simulink model "DriveSystemControl"  (R2023b)
settings: Solver=FixedStepAuto  StartTime=0.0  StopTime=Inf  FixedStep=0.001  RelTol=1e-3
PostLoadFcn:
  | if any(exist('dsrtsu_mdlpostloadfcn', 'file') ~= 0), dsrtsu_mdlpostloadfcn('Execute', bdroot); end
InitFcn:
  | , if any(exist('rtifpga_mdlclblib', 'file') ~= 0), rtifpga_mdlclblib('Init', bdroot); end,
  | , if any(exist('dsmpb_private', 'file') ~= 0), dsmpb_private('dsmpb_mdlclblib', 'Init', bdroot); end,
libraries: dsmpblib x2
(part 9 of 11)

== system DriveSystemControl/Bus Configuration (1) - Out/Manipulation/Virya Controller CAN File 08082024/WIP/CANChannel/PDUs/BMS02/sigBatteryCurrent/Feature Switch ==
  Feature Switch : Inport
  Term_sigBatteryCurrent Current Countdown Value : Terminator
  Term_sigBatteryCurrent Selected Feature : Terminator
  _Feature Switch_ : BusSelector  OutputSignals=sigBatteryCurrent Current Countdown Value,sigBatteryCurrent Selected Feature
  wires:
  Feature Switch/1 -> _Feature Switch_/1  "Feature Switch"
  _Feature Switch_/1 -> Term_sigBatteryCurrent Current Countdown Value/1  "<sigBatteryCurrent Current Countdown Value>"
  _Feature Switch_/2 -> Term_sigBatteryCurrent Selected Feature/1  "<sigBatteryCurrent Selected Feature>"

== system DriveSystemControl/Bus Configuration (1) - Out/Manipulation/Virya Controller CAN File 08082024/WIP/CANChannel/PDUs/BMS02/sigDriveCurrentLimit/Feature Switch ==
  Feature Switch : Inport
  Term_sigDriveCurrentLimit Current Countdown Value : Terminator
  Term_sigDriveCurrentLimit Selected Feature : Terminator
  _Feature Switch_ : BusSelector  OutputSignals=sigDriveCurrentLimit Current Countdown Value,sigDriveCurrentLimit Selected Feature
  wires:
  Feature Switch/1 -> _Feature Switch_/1  "Feature Switch"
  _Feature Switch_/1 -> Term_sigDriveCurrentLimit Current Countdown Value/1  "<sigDriveCurrentLimit Current Countdown Value>"
  _Feature Switch_/2 -> Term_sigDriveCurrentLimit Selected Feature/1  "<sigDriveCurrentLimit Selected Feature>"

== system DriveSystemControl/Bus Configuration (1) - Out/Manipulation/Virya Controller CAN File 08082024/WIP/CANChannel/PDUs/BMS02/sigRegenCurrentLimit/Feature Switch ==
  Feature Switch : Inport
  Term_sigRegenCurrentLimit Current Countdown Value : Terminator
  Term_sigRegenCurrentLimit Selected Feature : Terminator
  _Feature Switch_ : BusSelector  OutputSignals=sigRegenCurrentLimit Current Countdown Value,sigRegenCurrentLimit Selected Feature
  wires:
  Feature Switch/1 -> _Feature Switch_/1  "Feature Switch"
  _Feature Switch_/1 -> Term_sigRegenCurrentLimit Current Countdown Value/1  "<sigRegenCurrentLimit Current Countdown Value>"
  _Feature Switch_/2 -> Term_sigRegenCurrentLimit Selected Feature/1  "<sigRegenCurrentLimit Selected Feature>"

== system DriveSystemControl/Bus Configuration (1) - Out/Manipulation/Virya Controller CAN File 08082024/WIP/CANChannel/PDUs/BMS02/sigVehicleModeRequest/Feature Switch ==
  Feature Switch : Inport
  Term_sigVehicleModeRequest Current Countdown Value : Terminator
  Term_sigVehicleModeRequest Selected Feature : Terminator
  _Feature Switch_ : BusSelector  OutputSignals=sigVehicleModeRequest Current Countdown Value,sigVehicleModeRequest Selected Feature
  wires:
  Feature Switch/1 -> _Feature Switch_/1  "Feature Switch"
  _Feature Switch_/1 -> Term_sigVehicleModeRequest Current Countdown Value/1  "<sigVehicleModeRequest Current Countdown Value>"
  _Feature Switch_/2 -> Term_sigVehicleModeRequest Selected Feature/1  "<sigVehicleModeRequest Selected Feature>"

== system DriveSystemControl/Bus Configuration (1) - Out/Manipulation/Virya Controller CAN File 08082024/WIP/CANChannel/PDUs/MainController/CCU_heartBeat/Feature Switch ==
  Feature Switch : Inport
  Term_CCU_heartBeat Current Countdown Value : Terminator
  Term_CCU_heartBeat Selected Feature : Terminator
  _Feature Switch_ : BusSelector  OutputSignals=CCU_heartBeat Current Countdown Value,CCU_heartBeat Selected Feature
  wires:
  Feature Switch/1 -> _Feature Switch_/1  "Feature Switch"
  _Feature Switch_/1 -> Term_CCU_heartBeat Current Countdown Value/1  "<CCU_heartBeat Current Countdown Value>"
  _Feature Switch_/2 -> Term_CCU_heartBeat Selected Feature/1  "<CCU_heartBeat Selected Feature>"

== system DriveSystemControl/Bus Configuration (1) - Out/Manipulation/Virya Controller CAN File 08082024/WIP/CANChannel/PDUs/MainController/notUsed/Feature Switch ==
  Feature Switch : Inport
  Term_notUsed Current Countdown Value : Terminator
  Term_notUsed Selected Feature : Terminator
  _Feature Switch_ : BusSelector  OutputSignals=notUsed Current Countdown Value,notUsed Selected Feature
  wires:
  Feature Switch/1 -> _Feature Switch_/1  "Feature Switch"
  _Feature Switch_/1 -> Term_notUsed Current Countdown Value/1  "<notUsed Current Countdown Value>"
  _Feature Switch_/2 -> Term_notUsed Selected Feature/1  "<notUsed Selected Feature>"

== system DriveSystemControl/Bus Configuration (1) - Out/Manipulation/Virya Controller CAN File 08082024/WIP/CANChannel/PDUs/MainController/setAutoParkBreak/Feature Switch ==
  Feature Switch : Inport
  Term_setAutoParkBreak Current Countdown Value : Terminator
  Term_setAutoParkBreak Selected Feature : Terminator
  _Feature Switch_ : BusSelector  OutputSignals=setAutoParkBreak Current Countdown Value,setAutoParkBreak Selected Feature
  wires:
  Feature Switch/1 -> _Feature Switch_/1  "Feature Switch"
  _Feature Switch_/1 -> Term_setAutoParkBreak Current Countdown Value/1  "<setAutoParkBreak Current Countdown Value>"
  _Feature Switch_/2 -> Term_setAutoParkBreak Selected Feature/1  "<setAutoParkBreak Selected Feature>"

== system DriveSystemControl/Bus Configuration (1) - Out/Manipulation/Virya Controller CAN File 08082024/WIP/CANChannel/PDUs/MainController/setBreake/Feature Switch ==
  Feature Switch : Inport
  Term_setBreake Current Countdown Value : Terminator
  Term_setBreake Selected Feature : Terminator
  _Feature Switch_ : BusSelector  OutputSignals=setBreake Current Countdown Value,setBreake Selected Feature
  wires:
  Feature Switch/1 -> _Feature Switch_/1  "Feature Switch"
  _Feature Switch_/1 -> Term_setBreake Current Countdown Value/1  "<setBreake Current Countdown Value>"
  _Feature Switch_/2 -> Term_setBreake Selected Feature/1  "<setBreake Selected Feature>"

== system DriveSystemControl/Bus Configuration (1) - Out/Manipulation/Virya Controller CAN File 08082024/WIP/CANChannel/PDUs/MainController/setDirection/Feature Switch ==
  Feature Switch : Inport
  Term_setDirection Current Countdown Value : Terminator
  Term_setDirection Selected Feature : Terminator
  _Feature Switch_ : BusSelector  OutputSignals=setDirection Current Countdown Value,setDirection Selected Feature
  wires:
  Feature Switch/1 -> _Feature Switch_/1  "Feature Switch"
  _Feature Switch_/1 -> Term_setDirection Current Countdown Value/1  "<setDirection Current Countdown Value>"
  _Feature Switch_/2 -> Term_setDirection Selected Feature/1  "<setDirection Selected Feature>"

== system DriveSystemControl/Bus Configuration (1) - Out/Manipulation/Virya Controller CAN File 08082024/WIP/CANChannel/PDUs/MainController/setDriveMode/Feature Switch ==
  Feature Switch : Inport
  Term_setDriveMode Current Countdown Value : Terminator
  Term_setDriveMode Selected Feature : Terminator
  _Feature Switch_ : BusSelector  OutputSignals=setDriveMode Current Countdown Value,setDriveMode Selected Feature
  wires:
  Feature Switch/1 -> _Feature Switch_/1  "Feature Switch"
  _Feature Switch_/1 -> Term_setDriveMode Current Countdown Value/1  "<setDriveMode Current Countdown Value>"
  _Feature Switch_/2 -> Term_setDriveMode Selected Feature/1  "<setDriveMode Selected Feature>"

== system DriveSystemControl/Bus Configuration (1) - Out/Manipulation/Virya Controller CAN File 08082024/WIP/CANChannel/PDUs/MainController/setVelocity/Feature Switch ==
  Feature Switch : Inport
  Term_setVelocity Current Countdown Value : Terminator
  Term_setVelocity Selected Feature : Terminator
  _Feature Switch_ : BusSelector  OutputSignals=setVelocity Current Countdown Value,setVelocity Selected Feature
  wires:
  Feature Switch/1 -> _Feature Switch_/1  "Feature Switch"
  _Feature Switch_/1 -> Term_setVelocity Current Countdown Value/1  "<setVelocity Current Countdown Value>"
  _Feature Switch_/2 -> Term_setVelocity Selected Feature/1  "<setVelocity Selected Feature>"

== system DriveSystemControl/Bus Configuration (1) - Out/Manipulation/Virya Controller CAN File 08082024/WIP/CANChannel/PDUs/MainController/steeringPower/Feature Switch ==
  Feature Switch : Inport
  Term_steeringPower Current Countdown Value : Terminator
  Term_steeringPower Selected Feature : Terminator
  _Feature Switch_ : BusSelector  OutputSignals=steeringPower Current Countdown Value,steeringPower Selected Feature
  wires:
  Feature Switch/1 -> _Feature Switch_/1  "Feature Switch"
  _Feature Switch_/1 -> Term_steeringPower Current Countdown Value/1  "<steeringPower Current Countdown Value>"
  _Feature Switch_/2 -> Term_steeringPower Selected Feature/1  "<steeringPower Selected Feature>"

== system DriveSystemControl/Bus Configuration (1) - Out/Manipulation/Virya Controller CAN File 08082024/WIP/CANChannel/PDUs/TCU01/sigBrake/Feature Switch ==
  Feature Switch : Inport
  Term_sigBrake Current Countdown Value : Terminator
  Term_sigBrake Selected Feature : Terminator
  _Feature Switch_ : BusSelector  OutputSignals=sigBrake Current Countdown Value,sigBrake Selected Feature
  wires:
  Feature Switch/1 -> _Feature Switch_/1  "Feature Switch"
  _Feature Switch_/1 -> Term_sigBrake Current Countdown Value/1  "<sigBrake Current Countdown Value>"
  _Feature Switch_/2 -> Term_sigBrake Selected Feature/1  "<sigBrake Selected Feature>"

== system DriveSystemControl/Bus Configuration (1) - Out/Manipulation/Virya Controller CAN File 08082024/WIP/CANChannel/PDUs/TCU01/sigControllerTemperature/Feature Switch ==
  Feature Switch : Inport
  Term_sigControllerTemperature Current Countdown Value : Terminator
  Term_sigControllerTemperature Selected Feature : Terminator
  _Feature Switch_ : BusSelector  OutputSignals=sigControllerTemperature Current Countdown Value,sigControllerTemperature Selected Feature
  wires:
  Feature Switch/1 -> _Feature Switch_/1  "Feature Switch"
  _Feature Switch_/1 -> Term_sigControllerTemperature Current Countdown Value/1  "<sigControllerTemperature Current Countdown Value>"
  _Feature Switch_/2 -> Term_sigControllerTemperature Selected Feature/1  "<sigControllerTemperature Selected Feature>"

== system DriveSystemControl/Bus Configuration (1) - Out/Manipulation/Virya Controller CAN File 08082024/WIP/CANChannel/PDUs/TCU01/sigDriveMode/Feature Switch ==
  Feature Switch : Inport
  Term_sigDriveMode Current Countdown Value : Terminator
  Term_sigDriveMode Selected Feature : Terminator
  _Feature Switch_ : BusSelector  OutputSignals=sigDriveMode Current Countdown Value,sigDriveMode Selected Feature
  wires:
  Feature Switch/1 -> _Feature Switch_/1  "Feature Switch"
  _Feature Switch_/1 -> Term_sigDriveMode Current Countdown Value/1  "<sigDriveMode Current Countdown Value>"
  _Feature Switch_/2 -> Term_sigDriveMode Selected Feature/1  "<sigDriveMode Selected Feature>"

== system DriveSystemControl/Bus Configuration (1) - Out/Manipulation/Virya Controller CAN File 08082024/WIP/CANChannel/PDUs/TCU01/sigMotorTemperature/Feature Switch ==
  Feature Switch : Inport
  Term_sigMotorTemperature Current Countdown Value : Terminator
  Term_sigMotorTemperature Selected Feature : Terminator
  _Feature Switch_ : BusSelector  OutputSignals=sigMotorTemperature Current Countdown Value,sigMotorTemperature Selected Feature
  wires:
  Feature Switch/1 -> _Feature Switch_/1  "Feature Switch"
  _Feature Switch_/1 -> Term_sigMotorTemperature Current Countdown Value/1  "<sigMotorTemperature Current Countdown Value>"
  _Feature Switch_/2 -> Term_sigMotorTemperature Selected Feature/1  "<sigMotorTemperature Selected Feature>"

== system DriveSystemControl/Bus Configuration (1) - Out/Manipulation/Virya Controller CAN File 08082024/WIP/CANChannel/PDUs/TCU01/sigRMSCurrent/Feature Switch ==
  Feature Switch : Inport
  Term_sigRMSCurrent Current Countdown Value : Terminator
  Term_sigRMSCurrent Selected Feature : Terminator
  _Feature Switch_ : BusSelector  OutputSignals=sigRMSCurrent Current Countdown Value,sigRMSCurrent Selected Feature
  wires:
  Feature Switch/1 -> _Feature Switch_/1  "Feature Switch"
  _Feature Switch_/1 -> Term_sigRMSCurrent Current Countdown Value/1  "<sigRMSCurrent Current Countdown Value>"
  _Feature Switch_/2 -> Term_sigRMSCurrent Selected Feature/1  "<sigRMSCurrent Selected Feature>"

== system DriveSystemControl/Bus Configuration (1) - Out/Manipulation/Virya Controller CAN File 08082024/WIP/CANChannel/PDUs/TCU01/sigSpeed/Feature Switch ==
  Feature Switch : Inport
  Term_sigSpeed Current Countdown Value : Terminator
  Term_sigSpeed Selected Feature : Terminator
  _Feature Switch_ : BusSelector  OutputSignals=sigSpeed Current Countdown Value,sigSpeed Selected Feature
  wires:
  Feature Switch/1 -> _Feature Switch_/1  "Feature Switch"
  _Feature Switch_/1 -> Term_sigSpeed Current Countdown Value/1  "<sigSpeed Current Countdown Value>"
  _Feature Switch_/2 -> Term_sigSpeed Selected Feature/1  "<sigSpeed Selected Feature>"

== system DriveSystemControl/Bus Configuration (1) - Out/Manipulation/Virya Controller CAN File 08082024/WIP/CANChannel/PDUs/TCU01/sigThrottle/Feature Switch ==
  Feature Switch : Inport
  Term_sigThrottle Current Countdown Value : Terminator
  Term_sigThrottle Selected Feature : Terminator
  _Feature Switch_ : BusSelector  OutputSignals=sigThrottle Current Countdown Value,sigThrottle Selected Feature
  wires:
  Feature Switch/1 -> _Feature Switch_/1  "Feature Switch"
  _Feature Switch_/1 -> Term_sigThrottle Current Countdown Value/1  "<sigThrottle Current Countdown Value>"
  _Feature Switch_/2 -> Term_sigThrottle Selected Feature/1  "<sigThrottle Selected Feature>"

== system DriveSystemControl/Bus Configuration (1) - Out/Manipulation/Virya Controller CAN File 08082024/WIP/CANChannel/PDUs/TCU02/sigCapacitorVoltage/Feature Switch ==
  Feature Switch : Inport
  Term_sigCapacitorVoltage Current Countdown Value : Terminator
  Term_sigCapacitorVoltage Selected Feature : Terminator
  _Feature Switch_ : BusSelector  OutputSignals=sigCapacitorVoltage Current Countdown Value,sigCapacitorVoltage Selected Feature
  wires:
  Feature Switch/1 -> _Feature Switch_/1  "Feature Switch"
  _Feature Switch_/1 -> Term_sigCapacitorVoltage Current Countdown Value/1  "<sigCapacitorVoltage Current Countdown Value>"
  _Feature Switch_/2 -> Term_sigCapacitorVoltage Selected Feature/1  "<sigCapacitorVoltage Selected Feature>"

== system DriveSystemControl/Bus Configuration (1) - Out/Manipulation/Virya Controller CAN File 08082024/WIP/CANChannel/PDUs/TCU02/sigMotorRPM/Feature Switch ==
  Feature Switch : Inport
  Term_sigMotorRPM Current Countdown Value : Terminator
  Term_sigMotorRPM Selected Feature : Terminator
  _Feature Switch_ : BusSelector  OutputSignals=sigMotorRPM Current Countdown Value,sigMotorRPM Selected Feature
  wires:
  Feature Switch/1 -> _Feature Switch_/1  "Feature Switch"
  _Feature Switch_/1 -> Term_sigMotorRPM Current Countdown Value/1  "<sigMotorRPM Current Countdown Value>"
  _Feature Switch_/2 -> Term_sigMotorRPM Selected Feature/1  "<sigMotorRPM Selected Feature>"

== system DriveSystemControl/Bus Configuration (1) - Out/Manipulation/Virya Controller CAN File 08082024/WIP/CANChannel/PDUs/TCU02/sigOdometer/Feature Switch ==
  Feature Switch : Inport
  Term_sigOdometer Current Countdown Value : Terminator
  Term_sigOdometer Selected Feature : Terminator
  _Feature Switch_ : BusSelector  OutputSignals=sigOdometer Current Countdown Value,sigOdometer Selected Feature
  wires:
  Feature Switch/1 -> _Feature Switch_/1  "Feature Switch"
  _Feature Switch_/1 -> Term_sigOdometer Current Countdown Value/1  "<sigOdometer Current Countdown Value>"
  _Feature Switch_/2 -> Term_sigOdometer Selected Feature/1  "<sigOdometer Selected Feature>"

== system DriveSystemControl/Bus Configuration (1) - Out/Manipulation/Virya Controller CAN File 08082024/WIP/CANChannel/PDUs/TCU03/Controller_CompleteFaults/Feature Switch ==
  Feature Switch : Inport
  Term_Controller_CompleteFaults Current Countdown Value : Terminator
  Term_Controller_CompleteFaults Selected Feature : Terminator
  _Feature Switch_ : BusSelector  OutputSignals=Controller_CompleteFaults Current Countdown Value,Controller_CompleteFaults Selected Feature
  wires:
  Feature Switch/1 -> _Feature Switch_/1  "Feature Switch"
  _Feature Switch_/1 -> Term_Controller_CompleteFaults Current Countdown Value/1  "<Controller_CompleteFaults Current Countdown Value>"
  _Feature Switch_/2 -> Term_Controller_CompleteFaults Selected Feature/1  "<Controller_CompleteFaults Selected Feature>"

== system DriveSystemControl/Bus Configuration (1) - Out/Manipulation/Virya Controller CAN File 08082024/WIP/CANChannel/PDUs/TCU03/sig5VSupplyFailure/Feature Switch ==
  Feature Switch : Inport
  Term_sig5VSupplyFailure Current Countdown Value : Terminator
  Term_sig5VSupplyFailure Selected Feature : Terminator
  _Feature Switch_ : BusSelector  OutputSignals=sig5VSupplyFailure Current Countdown Value,sig5VSupplyFailure Selected Feature
  wires:
  Feature Switch/1 -> _Feature Switch_/1  "Feature Switch"
  _Feature Switch_/1 -> Term_sig5VSupplyFailure Current Countdown Value/1  "<sig5VSupplyFailure Current Countdown Value>"
  _Feature Switch_/2 -> Term_sig5VSupplyFailure Selected Feature/1  "<sig5VSupplyFailure Selected Feature>"

== system DriveSystemControl/Bus Configuration (1) - Out/Manipulation/Virya Controller CAN File 08082024/WIP/CANChannel/PDUs/TCU03/sigBPosOvervoltageCutback/Feature Switch ==
  Feature Switch : Inport
  Term_sigBPosOvervoltageCutback Current Countdown Value : Terminator
  Term_sigBPosOvervoltageCutback Selected Feature : Terminator
  _Feature Switch_ : BusSelector  OutputSignals=sigBPosOvervoltageCutback Current Countdown Value,sigBPosOvervoltageCutback Selected Feature
  wires:
  Feature Switch/1 -> _Feature Switch_/1  "Feature Switch"
  _Feature Switch_/1 -> Term_sigBPosOvervoltageCutback Current Countdown Value/1  "<sigBPosOvervoltageCutback Current Countdown Value>"
  _Feature Switch_/2 -> Term_sigBPosOvervoltageCutback Selected Feature/1  "<sigBPosOvervoltageCutback Selected Feature>"

== system DriveSystemControl/Bus Configuration (1) - Out/Manipulation/Virya Controller CAN File 08082024/WIP/CANChannel/PDUs/TCU03/sigBPosUndervoltageCutback/Feature Switch ==
  Feature Switch : Inport
  Term_sigBPosUndervoltageCutback Current Countdown Value : Terminator
  Term_sigBPosUndervoltageCutback Selected Feature : Terminator
  _Feature Switch_ : BusSelector  OutputSignals=sigBPosUndervoltageCutback Current Countdown Value,sigBPosUndervoltageCutback Selected Feature
  wires:
  Feature Switch/1 -> _Feature Switch_/1  "Feature Switch"
  _Feature Switch_/1 -> Term_sigBPosUndervoltageCutback Current Countdown Value/1  "<sigBPosUndervoltageCutback Current Countdown Value>"
  _Feature Switch_/2 -> Term_sigBPosUndervoltageCutback Selected Feature/1  "<sigBPosUndervoltageCutback Selected Feature>"

== system DriveSystemControl/Bus Configuration (1) - Out/Manipulation/Virya Controller CAN File 08082024/WIP/CANChannel/PDUs/TCU03/sigBadCalibration/Feature Switch ==
  Feature Switch : Inport
  Term_sigBadCalibration Current Countdown Value : Terminator
  Term_sigBadCalibration Selected Feature : Terminator
  _Feature Switch_ : BusSelector  OutputSignals=sigBadCalibration Current Countdown Value,sigBadCalibration Selected Feature
  wires:
  Feature Switch/1 -> _Feature Switch_/1  "Feature Switch"
  _Feature Switch_/1 -> Term_sigBadCalibration Current Countdown Value/1  "<sigBadCalibration Current Countdown Value>"
  _Feature Switch_/2 -> Term_sigBadCalibration Selected Feature/1  "<sigBadCalibration Selected Feature>"

== system DriveSystemControl/Bus Configuration (1) - Out/Manipulation/Virya Controller CAN File 08082024/WIP/CANChannel/PDUs/TCU03/sigBrakeWiperHigh/Feature Switch ==
  Feature Switch : Inport
  Term_sigBrakeWiperHigh Current Countdown Value : Terminator
  Term_sigBrakeWiperHigh Selected Feature : Terminator
  _Feature Switch_ : BusSelector  OutputSignals=sigBrakeWiperHigh Current Countdown Value,sigBrakeWiperHigh Selected Feature
  wires:
  Feature Switch/1 -> _Feature Switch_/1  "Feature Switch"
  _Feature Switch_/1 -> Term_sigBrakeWiperHigh Current Countdown Value/1  "<sigBrakeWiperHigh Current Countdown Value>"
  _Feature Switch_/2 -> Term_sigBrakeWiperHigh Selected Feature/1  "<sigBrakeWiperHigh Selected Feature>"

== system DriveSystemControl/Bus Configuration (1) - Out/Manipulation/Virya Controller CAN File 08082024/WIP/CANChannel/PDUs/TCU03/sigBrakeWiperLow/Feature Switch ==
  Feature Switch : Inport
  Term_sigBrakeWiperLow Current Countdown Value : Terminator
  Term_sigBrakeWiperLow Selected Feature : Terminator
  _Feature Switch_ : BusSelector  OutputSignals=sigBrakeWiperLow Current Countdown Value,sigBrakeWiperLow Selected Feature
  wires:
  Feature Switch/1 -> _Feature Switch_/1  "Feature Switch"
  _Feature Switch_/1 -> Term_sigBrakeWiperLow Current Countdown Value/1  "<sigBrakeWiperLow Current Countdown Value>"
  _Feature Switch_/2 -> Term_sigBrakeWiperLow Selected Feature/1  "<sigBrakeWiperLow Selected Feature>"

== system DriveSystemControl/Bus Configuration (1) - Out/Manipulation/Virya Controller CAN File 08082024/WIP/CANChannel/PDUs/TCU03/sigCoil2DriverOpenShort/Feature Switch ==
  Feature Switch : Inport
  Term_sigCoil2DriverOpenShort Current Countdown Value : Terminator
  Term_sigCoil2DriverOpenShort Selected Feature : Terminator
  _Feature Switch_ : BusSelector  OutputSignals=sigCoil2DriverOpenShort Current Countdown Value,sigCoil2DriverOpenShort Selected Feature
  wires:
  Feature Switch/1 -> _Feature Switch_/1  "Feature Switch"
  _Feature Switch_/1 -> Term_sigCoil2DriverOpenShort Current Countdown Value/1  "<sigCoil2DriverOpenShort Current Countdown Value>"
  _Feature Switch_/2 -> Term_sigCoil2DriverOpenShort Selected Feature/1  "<sigCoil2DriverOpenShort Selected Feature>"

== system DriveSystemControl/Bus Configuration (1) - Out/Manipulation/Virya Controller CAN File 08082024/WIP/CANChannel/PDUs/TCU03/sigCoil3DriverOpenShort/Feature Switch ==
  Feature Switch : Inport
  Term_sigCoil3DriverOpenShort Current Countdown Value : Terminator
  Term_sigCoil3DriverOpenShort Selected Feature : Terminator
  _Feature Switch_ : BusSelector  OutputSignals=sigCoil3DriverOpenShort Current Countdown Value,sigCoil3DriverOpenShort Selected Feature
  wires:
  Feature Switch/1 -> _Feature Switch_/1  "Feature Switch"
  _Feature Switch_/1 -> Term_sigCoil3DriverOpenShort Current Countdown Value/1  "<sigCoil3DriverOpenShort Current Countdown Value>"
  _Feature Switch_/2 -> Term_sigCoil3DriverOpenShort Selected Feature/1  "<sigCoil3DriverOpenShort Selected Feature>"

== system DriveSystemControl/Bus Configuration (1) - Out/Manipulation/Virya Controller CAN File 08082024/WIP/CANChannel/PDUs/TCU03/sigCoil4DriverOpenShort/Feature Switch ==
  Feature Switch : Inport
  Term_sigCoil4DriverOpenShort Current Countdown Value : Terminator
  Term_sigCoil4DriverOpenShort Selected Feature : Terminator
  _Feature Switch_ : BusSelector  OutputSignals=sigCoil4DriverOpenShort Current Countdown Value,sigCoil4DriverOpenShort Selected Feature
  wires:
  Feature Switch/1 -> _Feature Switch_/1  "Feature Switch"
  _Feature Switch_/1 -> Term_sigCoil4DriverOpenShort Current Countdown Value/1  "<sigCoil4DriverOpenShort Current Countdown Value>"
  _Feature Switch_/2 -> Term_sigCoil4DriverOpenShort Selected Feature/1  "<sigCoil4DriverOpenShort Selected Feature>"

== system DriveSystemControl/Bus Configuration (1) - Out/Manipulation/Virya Controller CAN File 08082024/WIP/CANChannel/PDUs/TCU03/sigControllerCommonFault/Feature Switch ==
  Feature Switch : Inport
  Term_sigControllerCommonFault Current Countdown Value : Terminator
  Term_sigControllerCommonFault Selected Feature : Terminator
  _Feature Switch_ : BusSelector  OutputSignals=sigControllerCommonFault Current Countdown Value,sigControllerCommonFault Selected Feature
  wires:
  Feature Switch/1 -> _Feature Switch_/1  "Feature Switch"
  _Feature Switch_/1 -> Term_sigControllerCommonFault Current Countdown Value/1  "<sigControllerCommonFault Current Countdown Value>"
  _Feature Switch_/2 -> Term_sigControllerCommonFault Selected Feature/1  "<sigControllerCommonFault Selected Feature>"

== system DriveSystemControl/Bus Configuration (1) - Out/Manipulation/Virya Controller CAN File 08082024/WIP/CANChannel/PDUs/TCU03/sigControllerOverCurrent/Feature Switch ==
  Feature Switch : Inport
  Term_sigControllerOverCurrent Current Countdown Value : Terminator
  Term_sigControllerOverCurrent Selected Feature : Terminator
  _Feature Switch_ : BusSelector  OutputSignals=sigControllerOverCurrent Current Countdown Value,sigControllerOverCurrent Selected Feature
  wires:
  Feature Switch/1 -> _Feature Switch_/1  "Feature Switch"
  _Feature Switch_/1 -> Term_sigControllerOverCurrent Current Countdown Value/1  "<sigControllerOverCurrent Current Countdown Value>"
  _Feature Switch_/2 -> Term_sigControllerOverCurrent Selected Feature/1  "<sigControllerOverCurrent Selected Feature>"

== system DriveSystemControl/Bus Configuration (1) - Out/Manipulation/Virya Controller CAN File 08082024/WIP/CANChannel/PDUs/TCU03/sigControllerOvertempCutback/Feature Switch ==
  Feature Switch : Inport
  Term_sigControllerOvertempCutback Current Countdown Value : Terminator
  Term_sigControllerOvertempCutback Selected Feature : Terminator
  _Feature Switch_ : BusSelector  OutputSignals=sigControllerOvertempCutback Current Countdown Value,sigControllerOvertempCutback Selected Feature
  wires:
  Feature Switch/1 -> _Feature Switch_/1  "Feature Switch"
  _Feature Switch_/1 -> Term_sigControllerOvertempCutback Current Countdown Value/1  "<sigControllerOvertempCutback Current Countdown Value>"
  _Feature Switch_/2 -> Term_sigControllerOvertempCutback Selected Feature/1  "<sigControllerOvertempCutback Selected Feature>"

== system DriveSystemControl/Bus Configuration (1) - Out/Manipulation/Virya Controller CAN File 08082024/WIP/CANChannel/PDUs/TCU03/sigControllerSevereOvertemp/Feature Switch ==
  Feature Switch : Inport
  Term_sigControllerSevereOvertemp Current Countdown Value : Terminator
  Term_sigControllerSevereOvertemp Selected Feature : Terminator
  _Feature Switch_ : BusSelector  OutputSignals=sigControllerSevereOvertemp Current Countdown Value,sigControllerSevereOvertemp Selected Feature
  wires:
  Feature Switch/1 -> _Feature Switch_/1  "Feature Switch"
  _Feature Switch_/1 -> Term_sigControllerSevereOvertemp Current Countdown Value/1  "<sigControllerSevereOvertemp Current Countdown Value>"
  _Feature Switch_/2 -> Term_sigControllerSevereOvertemp Selected Feature/1  "<sigControllerSevereOvertemp Selected Feature>"

== system DriveSystemControl/Bus Configuration (1) - Out/Manipulation/Virya Controller CAN File 08082024/WIP/CANChannel/PDUs/TCU03/sigControllerSevereUndertemp/Feature Switch ==
  Feature Switch : Inport
  Term_sigControllerSevereUndertemp Current Countdown Value : Terminator
  Term_sigControllerSevereUndertemp Selected Feature : Terminator
  _Feature Switch_ : BusSelector  OutputSignals=sigControllerSevereUndertemp Current Countdown Value,sigControllerSevereUndertemp Selected Feature
  wires:
  Feature Switch/1 -> _Feature Switch_/1  "Feature Switch"
  _Feature Switch_/1 -> Term_sigControllerSevereUndertemp Current Countdown Value/1  "<sigControllerSevereUndertemp Current Countdown Value>"
  _Feature Switch_/2 -> Term_sigControllerSevereUndertemp Selected Feature/1  "<sigControllerSevereUndertemp Selected Feature>"

== system DriveSystemControl/Bus Configuration (1) - Out/Manipulation/Virya Controller CAN File 08082024/WIP/CANChannel/PDUs/TCU03/sigCurrentSensorFault/Feature Switch ==
  Feature Switch : Inport
  Term_sigCurrentSensorFault Current Countdown Value : Terminator
  Term_sigCurrentSensorFault Selected Feature : Terminator
  _Feature Switch_ : BusSelector  OutputSignals=sigCurrentSensorFault Current Countdown Value,sigCurrentSensorFault Selected Feature
  wires:
  Feature Switch/1 -> _Feature Switch_/1  "Feature Switch"
  _Feature Switch_/1 -> Term_sigCurrentSensorFault Current Countdown Value/1  "<sigCurrentSensorFault Current Countdown Value>"
  _Feature Switch_/2 -> Term_sigCurrentSensorFault Selected Feature/1  "<sigCurrentSensorFault Selected Feature>"

== system DriveSystemControl/Bus Configuration (1) - Out/Manipulation/Virya Controller CAN File 08082024/WIP/CANChannel/PDUs/TCU03/sigEEPROMFailure/Feature Switch ==
  Feature Switch : Inport
  Term_sigEEPROMFailure Current Countdown Value : Terminator
  Term_sigEEPROMFailure Selected Feature : Terminator
  _Feature Switch_ : BusSelector  OutputSignals=sigEEPROMFailure Current Countdown Value,sigEEPROMFailure Selected Feature
  wires:
  Feature Switch/1 -> _Feature Switch_/1  "Feature Switch"
  _Feature Switch_/1 -> Term_sigEEPROMFailure Current Countdown Value/1  "<sigEEPROMFailure Current Countdown Value>"
  _Feature Switch_/2 -> Term_sigEEPROMFailure Selected Feature/1  "<sigEEPROMFailure Selected Feature>"

== system DriveSystemControl/Bus Configuration (1) - Out/Manipulation/Virya Controller CAN File 08082024/WIP/CANChannel/PDUs/TCU03/sigHighPedalDisable/Feature Switch ==
  Feature Switch : Inport
  Term_sigHighPedalDisable Current Countdown Value : Terminator
  Term_sigHighPedalDisable Selected Feature : Terminator
  _Feature Switch_ : BusSelector  OutputSignals=sigHighPedalDisable Current Countdown Value,sigHighPedalDisable Selected Feature
  wires:
  Feature Switch/1 -> _Feature Switch_/1  "Feature Switch"
  _Feature Switch_/1 -> Term_sigHighPedalDisable Current Countdown Value/1  "<sigHighPedalDisable Current Countdown Value>"
  _Feature Switch_/2 -> Term_sigHighPedalDisable Selected Feature/1  "<sigHighPedalDisable Selected Feature>"

== system DriveSystemControl/Bus Configuration (1) - Out/Manipulation/Virya Controller CAN File 08082024/WIP/CANChannel/PDUs/TCU03/sigInsulationResistanceLow/Feature Switch ==
  Feature Switch : Inport
  Term_sigInsulationResistanceLow Current Countdown Value : Terminator
  Term_sigInsulationResistanceLow Selected Feature : Terminator
  _Feature Switch_ : BusSelector  OutputSignals=sigInsulationResistanceLow Current Countdown Value,sigInsulationResistanceLow Selected Feature
  wires:
  Feature Switch/1 -> _Feature Switch_/1  "Feature Switch"
  _Feature Switch_/1 -> Term_sigInsulationResistanceLow Current Countdown Value/1  "<sigInsulationResistanceLow Current Countdown Value>"
  _Feature Switch_/2 -> Term_sigInsulationResistanceLow Selected Feature/1  "<sigInsulationResistanceLow Selected Feature>"

== system DriveSystemControl/Bus Configuration (1) - Out/Manipulation/Virya Controller CAN File 08082024/WIP/CANChannel/PDUs/TCU03/sigMainContactorWelded/Feature Switch ==
  Feature Switch : Inport
  Term_sigMainContactorWelded Current Countdown Value : Terminator
  Term_sigMainContactorWelded Selected Feature : Terminator
  _Feature Switch_ : BusSelector  OutputSignals=sigMainContactorWelded Current Countdown Value,sigMainContactorWelded Selected Feature
  wires:
  Feature Switch/1 -> _Feature Switch_/1  "Feature Switch"
  _Feature Switch_/1 -> Term_sigMainContactorWelded Current Countdown Value/1  "<sigMainContactorWelded Current Countdown Value>"
  _Feature Switch_/2 -> Term_sigMainContactorWelded Selected Feature/1  "<sigMainContactorWelded Selected Feature>"

== system DriveSystemControl/Bus Configuration (1) - Out/Manipulation/Virya Controller CAN File 08082024/WIP/CANChannel/PDUs/TCU03/sigMainContactordidnotClose/Feature Switch ==
  Feature Switch : Inport
  Term_sigMainContactordidnotClose Current Countdown Value : Terminator
  Term_sigMainContactordidnotClose Selected Feature : Terminator
  _Feature Switch_ : BusSelector  OutputSignals=sigMainContactordidnotClose Current Countdown Value,sigMainContactordidnotClose Selected Feature
  wires:
  Feature Switch/1 -> _Feature Switch_/1  "Feature Switch"
  _Feature Switch_/1 -> Term_sigMainContactordidnotClose Current Countdown Value/1  "<sigMainContactordidnotClose Current Countdown Value>"
  _Feature Switch_/2 -> Term_sigMainContactordidnotClose Selected Feature/1  "<sigMainContactordidnotClose Selected Feature>"

== system DriveSystemControl/Bus Configuration (1) - Out/Manipulation/Virya Controller CAN File 08082024/WIP/CANChannel/PDUs/TCU03/sigMainOpenShort/Feature Switch ==
  Feature Switch : Inport
  Term_sigMainOpenShort Current Countdown Value : Terminator
  Term_sigMainOpenShort Selected Feature : Terminator
  _Feature Switch_ : BusSelector  OutputSignals=sigMainOpenShort Current Countdown Value,sigMainOpenShort Selected Feature
  wires:
  Feature Switch/1 -> _Feature Switch_/1  "Feature Switch"
  _Feature Switch_/1 -> Term_sigMainOpenShort Current Countdown Value/1  "<sigMainOpenShort Current Countdown Value>"
  _Feature Switch_/2 -> Term_sigMainOpenShort Selected Feature/1  "<sigMainOpenShort Selected Feature>"

== system DriveSystemControl/Bus Configuration (1) - Out/Manipulation/Virya Controller CAN File 08082024/WIP/CANChannel/PDUs/TCU03/sigMotorCharacterization/Feature Switch ==
  Feature Switch : Inport
  Term_sigMotorCharacterization Current Countdown Value : Terminator
  Term_sigMotorCharacterization Selected Feature : Terminator
  _Feature Switch_ : BusSelector  OutputSignals=sigMotorCharacterization Current Countdown Value,sigMotorCharacterization Selected Feature
  wires:
  Feature Switch/1 -> _Feature Switch_/1  "Feature Switch"
  _Feature Switch_/1 -> Term_sigMotorCharacterization Current Countdown Value/1  "<sigMotorCharacterization Current Countdown Value>"
  _Feature Switch_/2 -> Term_sigMotorCharacterization Selected Feature/1  "<sigMotorCharacterization Selected Feature>"

== system DriveSystemControl/Bus Configuration (1) - Out/Manipulation/Virya Controller CAN File 08082024/WIP/CANChannel/PDUs/TCU03/sigMotorPhaseOpen/Feature Switch ==
  Feature Switch : Inport
  Term_sigMotorPhaseOpen Current Countdown Value : Terminator
  Term_sigMotorPhaseOpen Selected Feature : Terminator
  _Feature Switch_ : BusSelector  OutputSignals=sigMotorPhaseOpen Current Countdown Value,sigMotorPhaseOpen Selected Feature
  wires:
  Feature Switch/1 -> _Feature Switch_/1  "Feature Switch"
  _Feature Switch_/1 -> Term_sigMotorPhaseOpen Current Countdown Value/1  "<sigMotorPhaseOpen Current Countdown Value>"
  _Feature Switch_/2 -> Term_sigMotorPhaseOpen Selected Feature/1  "<sigMotorPhaseOpen Selected Feature>"

== system DriveSystemControl/Bus Configuration (1) - Out/Manipulation/Virya Controller CAN File 08082024/WIP/CANChannel/PDUs/TCU03/sigMotorTempHotCutback/Feature Switch ==
  Feature Switch : Inport
  Term_sigMotorTempHotCutback Current Countdown Value : Terminator
  Term_sigMotorTempHotCutback Selected Feature : Terminator
  _Feature Switch_ : BusSelector  OutputSignals=sigMotorTempHotCutback Current Countdown Value,sigMotorTempHotCutback Selected Feature
  wires:
  Feature Switch/1 -> _Feature Switch_/1  "Feature Switch"
  _Feature Switch_/1 -> Term_sigMotorTempHotCutback Current Countdown Value/1  "<sigMotorTempHotCutback Current Countdown Value>"
  _Feature Switch_/2 -> Term_sigMotorTempHotCutback Selected Feature/1  "<sigMotorTempHotCutback Selected Feature>"

== system DriveSystemControl/Bus Configuration (1) - Out/Manipulation/Virya Controller CAN File 08082024/WIP/CANChannel/PDUs/TCU03/sigMotorTempSensorFault/Feature Switch ==
  Feature Switch : Inport
  Term_sigMotorTempSensorFault Current Countdown Value : Terminator
  Term_sigMotorTempSensorFault Selected Feature : Terminator
  _Feature Switch_ : BusSelector  OutputSignals=sigMotorTempSensorFault Current Countdown Value,sigMotorTempSensorFault Selected Feature
  wires:
  Feature Switch/1 -> _Feature Switch_/1  "Feature Switch"
  _Feature Switch_/1 -> Term_sigMotorTempSensorFault Current Countdown Value/1  "<sigMotorTempSensorFault Current Countdown Value>"
  _Feature Switch_/2 -> Term_sigMotorTempSensorFault Selected Feature/1  "<sigMotorTempSensorFault Selected Feature>"

== system DriveSystemControl/Bus Configuration (1) - Out/Manipulation/Virya Controller CAN File 08082024/WIP/CANChannel/PDUs/TCU03/sigOEM_BatterySTOPSignal/Feature Switch ==
  Feature Switch : Inport
  Term_sigOEM_BatterySTOPSignal Current Countdown Value : Terminator
  Term_sigOEM_BatterySTOPSignal Selected Feature : Terminator
  _Feature Switch_ : BusSelector  OutputSignals=sigOEM_BatterySTOPSignal Current Countdown Value,sigOEM_BatterySTOPSignal Selected Feature
  wires:
  Feature Switch/1 -> _Feature Switch_/1  "Feature Switch"
  _Feature Switch_/1 -> Term_sigOEM_BatterySTOPSignal Current Countdown Value/1  "<sigOEM_BatterySTOPSignal Current Countdown Value>"
  _Feature Switch_/2 -> Term_sigOEM_BatterySTOPSignal Selected Feature/1  "<sigOEM_BatterySTOPSignal Selected Feature>"

== system DriveSystemControl/Bus Configuration (1) - Out/Manipulation/Virya Controller CAN File 08082024/WIP/CANChannel/PDUs/TCU03/sigOEM_NoBatteryCAN/Feature Switch ==
  Feature Switch : Inport
  Term_sigOEM_NoBatteryCAN Current Countdown Value : Terminator
  Term_sigOEM_NoBatteryCAN Selected Feature : Terminator
  _Feature Switch_ : BusSelector  OutputSignals=sigOEM_NoBatteryCAN Current Countdown Value,sigOEM_NoBatteryCAN Selected Feature
  wires:
  Feature Switch/1 -> _Feature Switch_/1  "Feature Switch"
  _Feature Switch_/1 -> Term_sigOEM_NoBatteryCAN Current Countdown Value/1  "<sigOEM_NoBatteryCAN Current Countdown Value>"
  _Feature Switch_/2 -> Term_sigOEM_NoBatteryCAN Selected Feature/1  "<sigOEM_NoBatteryCAN Selected Feature>"

== system DriveSystemControl/Bus Configuration (1) - Out/Manipulation/Virya Controller CAN File 08082024/WIP/CANChannel/PDUs/TCU03/sigOSGeneral/Feature Switch ==
  Feature Switch : Inport
  Term_sigOSGeneral Current Countdown Value : Terminator
  Term_sigOSGeneral Selected Feature : Terminator
  _Feature Switch_ : BusSelector  OutputSignals=sigOSGeneral Current Countdown Value,sigOSGeneral Selected Feature
  wires:
  Feature Switch/1 -> _Feature Switch_/1  "Feature Switch"
  _Feature Switch_/1 -> Term_sigOSGeneral Current Countdown Value/1  "<sigOSGeneral Current Countdown Value>"
  _Feature Switch_/2 -> Term_sigOSGeneral Selected Feature/1  "<sigOSGeneral Selected Feature>"

== system DriveSystemControl/Bus Configuration (1) - Out/Manipulation/Virya Controller CAN File 08082024/WIP/CANChannel/PDUs/TCU03/sigPMACCommissioningNeeded/Feature Switch ==
  Feature Switch : Inport
  Term_sigPMACCommissioningNeeded Current Countdown Value : Terminator
  Term_sigPMACCommissioningNeeded Selected Feature : Terminator
  _Feature Switch_ : BusSelector  OutputSignals=sigPMACCommissioningNeeded Current Countdown Value,sigPMACCommissioningNeeded Selected Feature
  wires:
  Feature Switch/1 -> _Feature Switch_/1  "Feature Switch"
  _Feature Switch_/1 -> Term_sigPMACCommissioningNeeded Current Countdown Value/1  "<sigPMACCommissioningNeeded Current Countdown Value>"
  _Feature Switch_/2 -> Term_sigPMACCommissioningNeeded Selected Feature/1  "<sigPMACCommissioningNeeded Selected Feature>"

== system DriveSystemControl/Bus Configuration (1) - Out/Manipulation/Virya Controller CAN File 08082024/WIP/CANChannel/PDUs/TCU03/sigParameterChangeFault/Feature Switch ==
  Feature Switch : Inport
  Term_sigParameterChangeFault Current Countdown Value : Terminator
  Term_sigParameterChangeFault Selected Feature : Terminator
  _Feature Switch_ : BusSelector  OutputSignals=sigParameterChangeFault Current Countdown Value,sigParameterChangeFault Selected Feature
  wires:
  Feature Switch/1 -> _Feature Switch_/1  "Feature Switch"
  _Feature Switch_/1 -> Term_sigParameterChangeFault Current Countdown Value/1  "<sigParameterChangeFault Current Countdown Value>"
  _Feature Switch_/2 -> Term_sigParameterChangeFault Selected Feature/1  "<sigParameterChangeFault Selected Feature>"

== system DriveSystemControl/Bus Configuration (1) - Out/Manipulation/Virya Controller CAN File 08082024/WIP/CANChannel/PDUs/TCU03/sigPhasePWMMismatch/Feature Switch ==
  Feature Switch : Inport
  Term_sigPhasePWMMismatch Current Countdown Value : Terminator
  Term_sigPhasePWMMismatch Selected Feature : Terminator
  _Feature Switch_ : BusSelector  OutputSignals=sigPhasePWMMismatch Current Countdown Value,sigPhasePWMMismatch Selected Feature
  wires:
  Feature Switch/1 -> _Feature Switch_/1  "Feature Switch"
  _Feature Switch_/1 -> Term_sigPhasePWMMismatch Current Countdown Value/1  "<sigPhasePWMMismatch Current Countdown Value>"
  _Feature Switch_/2 -> Term_sigPhasePWMMismatch Selected Feature/1  "<sigPhasePWMMismatch Selected Feature>"

== system DriveSystemControl/Bus Configuration (1) - Out/Manipulation/Virya Controller CAN File 08082024/WIP/CANChannel/PDUs/TCU03/sigPrechargeFailed/Feature Switch ==
  Feature Switch : Inport
  Term_sigPrechargeFailed Current Countdown Value : Terminator
  Term_sigPrechargeFailed Selected Feature : Terminator
  _Feature Switch_ : BusSelector  OutputSignals=sigPrechargeFailed Current Countdown Value,sigPrechargeFailed Selected Feature
  wires:
  Feature Switch/1 -> _Feature Switch_/1  "Feature Switch"
  _Feature Switch_/1 -> Term_sigPrechargeFailed Current Countdown Value/1  "<sigPrechargeFailed Current Countdown Value>"
  _Feature Switch_/2 -> Term_sigPrechargeFailed Selected Feature/1  "<sigPrechargeFailed Selected Feature>"

== system DriveSystemControl/Bus Configuration (1) - Out/Manipulation/Virya Controller CAN File 08082024/WIP/CANChannel/PDUs/TCU03/sigSevereBPosOvervoltage/Feature Switch ==
  Feature Switch : Inport
  Term_sigSevereBPosOvervoltage Current Countdown Value : Terminator
  Term_sigSevereBPosOvervoltage Selected Feature : Terminator
  _Feature Switch_ : BusSelector  OutputSignals=sigSevereBPosOvervoltage Current Countdown Value,sigSevereBPosOvervoltage Selected Feature
  wires:
  Feature Switch/1 -> _Feature Switch_/1  "Feature Switch"
  _Feature Switch_/1 -> Term_sigSevereBPosOvervoltage Current Countdown Value/1  "<sigSevereBPosOvervoltage Current Countdown Value>"
  _Feature Switch_/2 -> Term_sigSevereBPosOvervoltage Selected Feature/1  "<sigSevereBPosOvervoltage Selected Feature>"

== system DriveSystemControl/Bus Configuration (1) - Out/Manipulation/Virya Controller CAN File 08082024/WIP/CANChannel/PDUs/TCU03/sigSevereBPosUndervoltage/Feature Switch ==
  Feature Switch : Inport
  Term_sigSevereBPosUndervoltage Current Countdown Value : Terminator
  Term_sigSevereBPosUndervoltage Selected Feature : Terminator
  _Feature Switch_ : BusSelector  OutputSignals=sigSevereBPosUndervoltage Current Countdown Value,sigSevereBPosUndervoltage Selected Feature
  wires:
  Feature Switch/1 -> _Feature Switch_/1  "Feature Switch"
  _Feature Switch_/1 -> Term_sigSevereBPosUndervoltage Current Countdown Value/1  "<sigSevereBPosUndervoltage Current Countdown Value>"
  _Feature Switch_/2 -> Term_sigSevereBPosUndervoltage Selected Feature/1  "<sigSevereBPosUndervoltage Selected Feature>"

== system DriveSystemControl/Bus Configuration (1) - Out/Manipulation/Virya Controller CAN File 08082024/WIP/CANChannel/PDUs/TCU03/sigSevereKSIOvervoltage/Feature Switch ==
  Feature Switch : Inport
  Term_sigSevereKSIOvervoltage Current Countdown Value : Terminator
  Term_sigSevereKSIOvervoltage Selected Feature : Terminator
  _Feature Switch_ : BusSelector  OutputSignals=sigSevereKSIOvervoltage Current Countdown Value,sigSevereKSIOvervoltage Selected Feature
  wires:
  Feature Switch/1 -> _Feature Switch_/1  "Feature Switch"
  _Feature Switch_/1 -> Term_sigSevereKSIOvervoltage Current Countdown Value/1  "<sigSevereKSIOvervoltage Current Countdown Value>"
  _Feature Switch_/2 -> Term_sigSevereKSIOvervoltage Selected Feature/1  "<sigSevereKSIOvervoltage Selected Feature>"

== system DriveSystemControl/Bus Configuration (1) - Out/Manipulation/Virya Controller CAN File 08082024/WIP/CANChannel/PDUs/TCU03/sigSevereKSIUndervoltage/Feature Switch ==
  Feature Switch : Inport
  Term_sigSevereKSIUndervoltage Current Countdown Value : Terminator
  Term_sigSevereKSIUndervoltage Selected Feature : Terminator
  _Feature Switch_ : BusSelector  OutputSignals=sigSevereKSIUndervoltage Current Countdown Value,sigSevereKSIUndervoltage Selected Feature
  wires:
  Feature Switch/1 -> _Feature Switch_/1  "Feature Switch"
  _Feature Switch_/1 -> Term_sigSevereKSIUndervoltage Current Countdown Value/1  "<sigSevereKSIUndervoltage Current Countdown Value>"
  _Feature Switch_/2 -> Term_sigSevereKSIUndervoltage Selected Feature/1  "<sigSevereKSIUndervoltage Selected Feature>"

== system DriveSystemControl/Bus Configuration (1) - Out/Manipulation/Virya Controller CAN File 08082024/WIP/CANChannel/PDUs/TCU03/sigSinCosMisalignment/Feature Switch ==
  Feature Switch : Inport
  Term_sigSinCosMisalignment Current Countdown Value : Terminator
  Term_sigSinCosMisalignment Selected Feature : Terminator
  _Feature Switch_ : BusSelector  OutputSignals=sigSinCosMisalignment Current Countdown Value,sigSinCosMisalignment Selected Feature
  wires:
  Feature Switch/1 -> _Feature Switch_/1  "Feature Switch"
  _Feature Switch_/1 -> Term_sigSinCosMisalignment Current Countdown Value/1  "<sigSinCosMisalignment Current Countdown Value>"
  _Feature Switch_/2 -> Term_sigSinCosMisalignment Selected Feature/1  "<sigSinCosMisalignment Selected Feature>"

== system DriveSystemControl/Bus Configuration (1) - Out/Manipulation/Virya Controller CAN File 08082024/WIP/CANChannel/PDUs/TCU03/sigSinCosSensorFault/Feature Switch ==
  Feature Switch : Inport
  Term_sigSinCosSensorFault Current Countdown Value : Terminator
  Term_sigSinCosSensorFault Selected Feature : Terminator
  _Feature Switch_ : BusSelector  OutputSignals=sigSinCosSensorFault Current Countdown Value,sigSinCosSensorFault Selected Feature
  wires:
  Feature Switch/1 -> _Feature Switch_/1  "Feature Switch"
  _Feature Switch_/1 -> Term_sigSinCosSensorFault Current Countdown Value/1  "<sigSinCosSensorFault Current Countdown Value>"
  _Feature Switch_/2 -> Term_sigSinCosSensorFault Selected Feature/1  "<sigSinCosSensorFault Selected Feature>"

== system DriveSystemControl/Bus Configuration (1) - Out/Manipulation/Virya Controller CAN File 08082024/WIP/CANChannel/PDUs/TCU03/sigStallDetected/Feature Switch ==
  Feature Switch : Inport
  Term_sigStallDetected Current Countdown Value : Terminator
  Term_sigStallDetected Selected Feature : Terminator
  _Feature Switch_ : BusSelector  OutputSignals=sigStallDetected Current Countdown Value,sigStallDetected Selected Feature
  wires:
  Feature Switch/1 -> _Feature Switch_/1  "Feature Switch"
  _Feature Switch_/1 -> Term_sigStallDetected Current Countdown Value/1  "<sigStallDetected Current Countdown Value>"
  _Feature Switch_/2 -> Term_sigStallDetected Selected Feature/1  "<sigStallDetected Selected Feature>"

== system DriveSystemControl/Bus Configuration (1) - Out/Manipulation/Virya Controller CAN File 08082024/WIP/CANChannel/PDUs/TCU03/sigSupervisorFault/Feature Switch ==
  Feature Switch : Inport
  Term_sigSupervisorFault Current Countdown Value : Terminator
  Term_sigSupervisorFault Selected Feature : Terminator
  _Feature Switch_ : BusSelector  OutputSignals=sigSupervisorFault Current Countdown Value,sigSupervisorFault Selected Feature
  wires:
  Feature Switch/1 -> _Feature Switch_/1  "Feature Switch"
  _Feature Switch_/1 -> Term_sigSupervisorFault Current Countdown Value/1  "<sigSupervisorFault Current Countdown Value>"
  _Feature Switch_/2 -> Term_sigSupervisorFault Selected Feature/1  "<sigSupervisorFault Selected Feature>"

== system DriveSystemControl/Bus Configuration (1) - Out/Manipulation/Virya Controller CAN File 08082024/WIP/CANChannel/PDUs/TCU03/sigThrottlewiperHigh/Feature Switch ==
  Feature Switch : Inport
  Term_sigThrottlewiperHigh Current Countdown Value : Terminator
  Term_sigThrottlewiperHigh Selected Feature : Terminator
  _Feature Switch_ : BusSelector  OutputSignals=sigThrottlewiperHigh Current Countdown Value,sigThrottlewiperHigh Selected Feature
  wires:
  Feature Switch/1 -> _Feature Switch_/1  "Feature Switch"
  _Feature Switch_/1 -> Term_sigThrottlewiperHigh Current Countdown Value/1  "<sigThrottlewiperHigh Current Countdown Value>"
  _Feature Switch_/2 -> Term_sigThrottlewiperHigh Selected Feature/1  "<sigThrottlewiperHigh Selected Feature>"

== system DriveSystemControl/Bus Configuration (1) - Out/Manipulation/Virya Controller CAN File 08082024/WIP/CANChannel/PDUs/TCU03/sigThrottlewiperLow/Feature Switch ==
  Feature Switch : Inport
  Term_sigThrottlewiperLow Current Countdown Value : Terminator
  Term_sigThrottlewiperLow Selected Feature : Terminator
  _Feature Switch_ : BusSelector  OutputSignals=sigThrottlewiperLow Current Countdown Value,sigThrottlewiperLow Selected Feature
  wires:
  Feature Switch/1 -> _Feature Switch_/1  "Feature Switch"
  _Feature Switch_/1 -> Term_sigThrottlewiperLow Current Countdown Value/1  "<sigThrottlewiperLow Current Countdown Value>"
  _Feature Switch_/2 -> Term_sigThrottlewiperLow Selected Feature/1  "<sigThrottlewiperLow Selected Feature>"

== system DriveSystemControl/Bus Configuration (1) - Out/Manipulation/Virya Controller CAN File 08082024/WIP/CANChannel/PDUs/TCU03/sigVCLRunTimeError/Feature Switch ==
  Feature Switch : Inport
  Term_sigVCLRunTimeError Current Countdown Value : Terminator
  Term_sigVCLRunTimeError Selected Feature : Terminator
  _Feature Switch_ : BusSelector  OutputSignals=sigVCLRunTimeError Current Countdown Value,sigVCLRunTimeError Selected Feature
  wires:
  Feature Switch/1 -> _Feature Switch_/1  "Feature Switch"
  _Feature Switch_/1 -> Term_sigVCLRunTimeError Current Countdown Value/1  "<sigVCLRunTimeError Current Countdown Value>"
  _Feature Switch_/2 -> Term_sigVCLRunTimeError Selected Feature/1  "<sigVCLRunTimeError Selected Feature>"
